simulink library "ComponentsLib"  (R2022b)
settings: Solver=VariableStepAuto  StartTime=0.0  StopTime=10.0  RelTol=1e-3
undefined symbols (not defined in the file or in its folder): SimIn, SimPar
libraries: simulink_extras x23, libAxisTransformations x2
settings Model: Creator=tbritton  LastModifiedBy=macheson
settings SolverCC: AlgebraicLoopSolver=TrustRegion
settings DebuggingCC: UnconnectedInputMsg=warning  UnconnectedOutputMsg=warning  UnconnectedLineMsg=warning  SFMachineParentedDataDiag=warning
settings ModelReferenceCC: EnableRefExpFcnMdlSchedulingChecks=on
settings RTWCC: DLArmComputeVersion=19.05

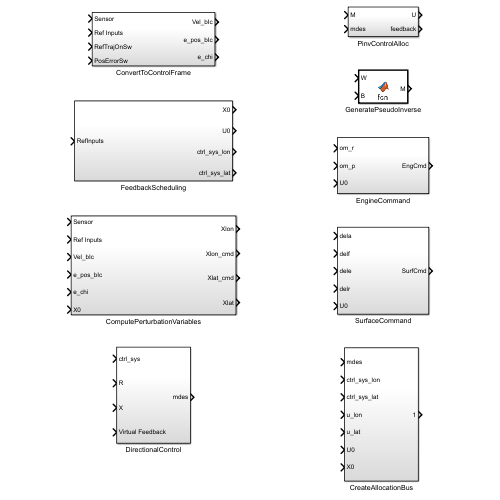
[thumbnail: Simulink's stored preview of the top-level diagram]
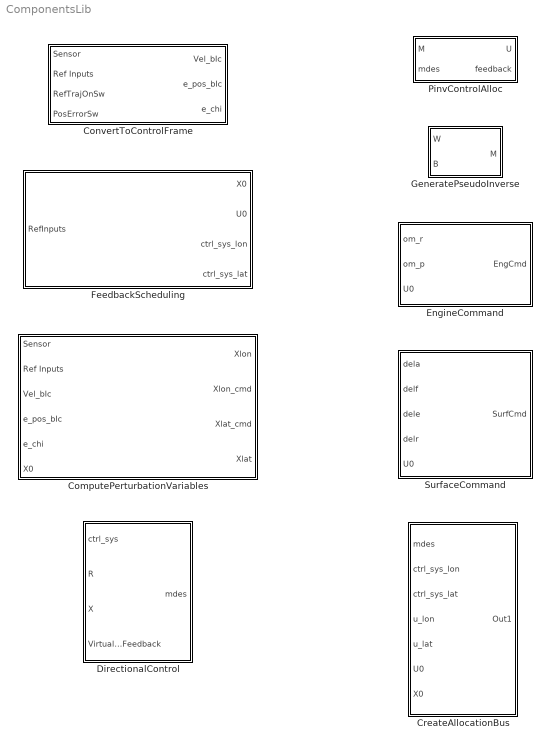
== system ComponentsLib ==
  ComputePerturbationVariables : Subsystem
  ConvertToControlFrame : Subsystem
  CreateAllocationBus : Subsystem
  DirectionalControl : Subsystem
  EngineCommand : Subsystem
  FeedbackScheduling : Subsystem
  GeneratePseudoInverse : MATLAB Function  TreatAsAtomicUnit=on
  PinvControlAlloc : Subsystem
  SurfaceCommand : Subsystem

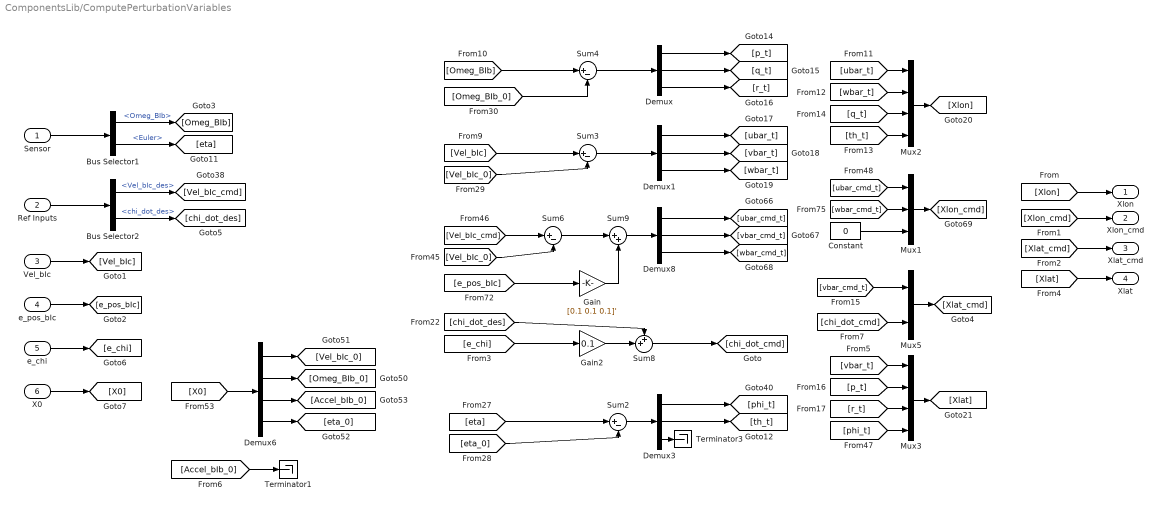
== system ComponentsLib/ComputePerturbationVariables ==
  Sensor : Inport  OutDataTypeStr=Bus: SensorBus
  Ref Inputs : Inport  Port=2  OutDataTypeStr=Bus: BUS_REF_INPUT
  Vel_bIc : Inport  Port=3
  e_pos_bIc : Inport  Port=4
  e_chi : Inport  Port=5
  X0 : Inport  Port=6
  Bus Selector1 : BusSelector  OutputSignals=Omeg_BIb,Euler
  Bus Selector2 : BusSelector  OutputSignals=Vel_bIc_des,chi_dot_des
  Constant : Constant  Value=0
  Demux{,1,3,8} (4 alike) : Demux  Outputs=3
  Demux6 : Demux  Outputs=[3 3 3 3]
  Gain : Gain  Gain=[0.1 0.1 0.1]'
  Gain2 : Gain  Gain=0.1
  Mux1 : Mux  Inputs=3
  Mux2 : Mux
  Mux3 : Mux
  Mux5 : Mux  Inputs=2
  Sum{2..4,6} (4 alike) : Sum  Inputs=|+-
  Sum8 : Sum  Inputs=++|
  Sum9 : Sum  Inputs=|++
  Terminator1 : Terminator
  Terminator3 : Terminator
  Xlon : Outport
  Xlon_cmd : Outport  Port=2
  Xlat_cmd : Outport  Port=3
  Xlat : Outport  Port=4
  wires:
  [Omeg_BIb_0] -> Sum4/2
  Sum9/1 -> Demux8/1
  [Vel_bIc] -> Sum3/1
  [Vel_bIc_0] -> Sum3/2
  [chi_dot_cmd] -> Mux5/2
  Demux1/1 -> [ubar_t]
  [eta] -> Sum2/1
  Demux3/2 -> [th_t]
  Demux3/3 -> Terminator3/1
  Demux3/1 -> [phi_t]
  Demux1/3 -> [wbar_t]
  Demux/1 -> [p_t]
  Gain2/1 -> Sum8/2
  Mux2/1 -> [Xlon]
  Sum8/1 -> [chi_dot_cmd]
  [e_chi] -> Gain2/1
  [Vel_bIc_0] -> Sum6/2
  [r_t] -> Mux3/3
  [vbar_cmd_t] -> Mux5/1
  Gain/1 -> Sum9/2
  [ubar_t] -> Mux2/1
  Mux5/1 -> [Xlat_cmd]
  [q_t] -> Mux2/3
  Demux1/2 -> [vbar_t]
  [chi_dot_des] -> Sum8/1
  Mux1/1 -> [Xlon_cmd]
  [vbar_t] -> Mux3/1
  [wbar_cmd_t] -> Mux1/2
  [e_pos_bIc] -> Gain/1
  Demux8/3 -> [wbar_cmd_t]
  Constant/1 -> Mux1/3
  [phi_t] -> Mux3/4
  Demux8/1 -> [ubar_cmd_t]
  Sum6/1 -> Sum9/1
  [Vel_bIc_cmd] -> Sum6/1
  Demux8/2 -> [vbar_cmd_t]
  Sum2/1 -> Demux3/1
  Demux/3 -> [r_t]
  Sum3/1 -> Demux1/1
  Sum4/1 -> Demux/1
  Mux3/1 -> [Xlat]
  [p_t] -> Mux3/2
  [th_t] -> Mux2/4
  Demux/2 -> [q_t]
  [ubar_cmd_t] -> Mux1/1
  [wbar_t] -> Mux2/2
  [eta_0] -> Sum2/2
  [Omeg_BIb] -> Sum4/1
  [Xlon] -> Xlon/1
  [Xlon_cmd] -> Xlon_cmd/1
  [Xlat_cmd] -> Xlat_cmd/1
  [Xlat] -> Xlat/1
  Bus Selector1/2 -> [eta]  "<Euler>"
  Sensor/1 -> Bus Selector1/1
  Bus Selector1/1 -> [Omeg_BIb]  "<Omeg_BIb>"
  Vel_bIc/1 -> [Vel_bIc]
  Ref Inputs/1 -> Bus Selector2/1
  Bus Selector2/1 -> [Vel_bIc_cmd]  "<Vel_bIc_des>"
  Bus Selector2/2 -> [chi_dot_des]  "<chi_dot_des>"
  e_pos_bIc/1 -> [e_pos_bIc]
  e_chi/1 -> [e_chi]
  Demux6/1 -> [Vel_bIc_0]
  Demux6/3 -> [Accel_bIb_0]
  [X0] -> Demux6/1
  Demux6/4 -> [eta_0]
  Demux6/2 -> [Omeg_BIb_0]
  X0/1 -> [X0]
  [Accel_bIb_0] -> Terminator1/1

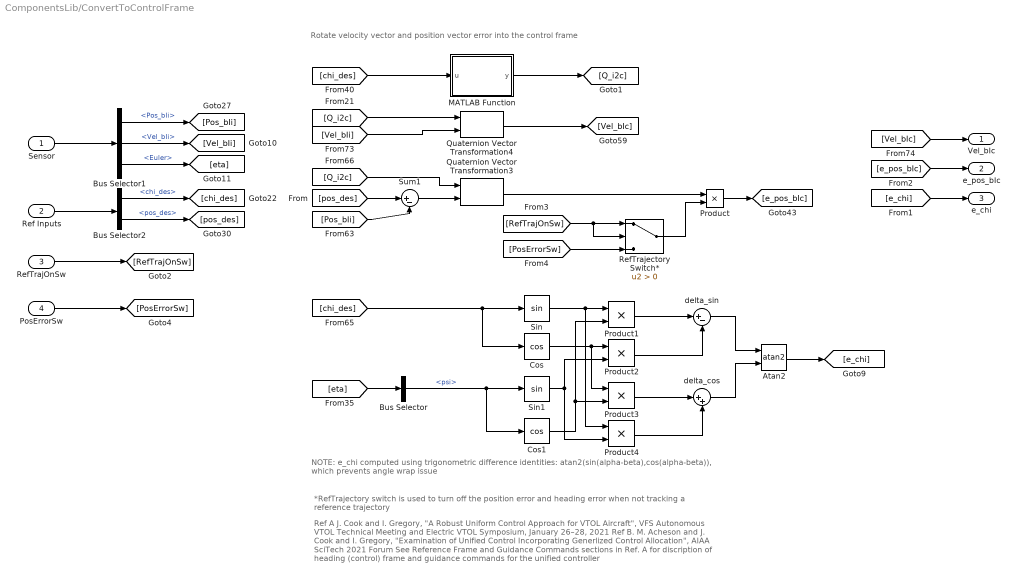
== system ComponentsLib/ConvertToControlFrame ==
  note: NOTE: e_chi computed using trigonometric difference identities: atan2(sin(alpha-beta),cos(alpha-beta)), which prevents angle wrap issue
  note: *RefTrajectory switch is used to turn off the position error and heading error when not tracking a reference trajectory
  note: Ref A
      | J. Cook and I. Gregory, "A Robust Uniform Control Approach for VTOL Aircraft", VFS Autonomous VTOL Technical Meeting and Electric VTOL Symposium, January 26–28, 2021
      |
      | Ref B.
      | M. Acheson and J. Cook and I. Gregory, "Examination of Unified Control Incorporating Generlized Control Allocation", AIAA SciTech 2021 Forum
      |
      | See Reference Frame and Guidance Commands sections in Ref. A for discription of heading (control) frame and guidance commands for the unified controller
  note: Rotate velocity vector and position vector error into the control frame
  Sensor : Inport  OutDataTypeStr=Bus: SensorBus
  Ref Inputs : Inport  Port=2  OutDataTypeStr=Bus: BUS_REF_INPUT
  RefTrajOnSw : Inport  Port=3
  PosErrorSw : Inport  Port=4
  Atan2 : Trigonometry  Operator=atan2
  Bus Selector : BusSelector  OutputSignals=psi
  Bus Selector1 : BusSelector  OutputSignals=Pos_bIi,Vel_bIi,Euler
  Bus Selector2 : BusSelector  OutputSignals=chi_des,pos_des
  Cos : Trigonometry  Operator=cos
  Cos1 : Trigonometry  Operator=cos
  MATLAB Function : MATLAB Function  TreatAsAtomicUnit=on
  Product{,1..4} (5 alike) : Product
  Quaternion Vector Transformation3 : libAxisTransformations/Quaternion Vector Transformation  n=0
  Quaternion Vector Transformation4 : libAxisTransformations/Quaternion Vector Transformation  n=0
  RefTrajectory Switch* : Switch  Criteria=u2 > Threshold  SaturateOnIntegerOverflow=off  InputSameDT=off
  Sin : Trigonometry
  Sin1 : Trigonometry
  Sum1 : Sum  Inputs=|+-
  delta_cos : Sum  Inputs=|++
  delta_sin : Sum  Inputs=|+-
  Vel_bIc : Outport
  e_pos_bIc : Outport  Port=2
  e_chi : Outport  Port=3
  wires:
  Sensor/1 -> Bus Selector1/1
  Quaternion Vector Transformation4/1 -> [Vel_bIc]
  [chi_des] -> Cos/1, Sin/1
  Sum1/1 -> Quaternion Vector Transformation3/2
  [e_pos_bIc] -> e_pos_bIc/1
  RefTrajOnSw/1 -> [RefTrajOnSw]
  Bus Selector2/1 -> [chi_des]  "<chi_des>"
  Bus Selector1/2 -> [Vel_bIi]  "<Vel_bIi>"
  PosErrorSw/1 -> [PosErrorSw]
  [Vel_bIi] -> Quaternion Vector Transformation4/2
  Atan2/1 -> [e_chi]
  Bus Selector1/1 -> [Pos_bIi]  "<Pos_bIi>"
  Bus Selector2/2 -> [pos_des]  "<pos_des>"
  [RefTrajOnSw] -> RefTrajectory Switch*/1, RefTrajectory Switch*/2
  [Vel_bIc] -> Vel_bIc/1
  [Pos_bIi] -> Sum1/2
  RefTrajectory Switch*/1 -> Product/2
  [chi_des] -> MATLAB Function/1(u)
  [e_chi] -> e_chi/1
  [pos_des] -> Sum1/1
  Quaternion Vector Transformation3/1 -> Product/1
  [Q_i2c] -> Quaternion Vector Transformation3/1
  Product/1 -> [e_pos_bIc]
  Ref Inputs/1 -> Bus Selector2/1
  MATLAB Function/1(y) -> [Q_i2c]
  Bus Selector1/3 -> [eta]  "<Euler>"
  [PosErrorSw] -> RefTrajectory Switch*/3
  [eta] -> Bus Selector/1
  [Q_i2c] -> Quaternion Vector Transformation4/1
  Bus Selector/1 -> Cos1/1, Sin1/1  "<psi>"
  Sin/1 -> Product1/1, Product4/1
  Cos/1 -> Product3/1, Product2/1
  Sin1/1 -> Product4/2, Product2/2
  Cos1/1 -> Product3/2, Product1/2
  Product1/1 -> delta_sin/1
  Product2/1 -> delta_sin/2
  Product3/1 -> delta_cos/1
  Product4/1 -> delta_cos/2
  delta_sin/1 -> Atan2/1
  delta_cos/1 -> Atan2/2

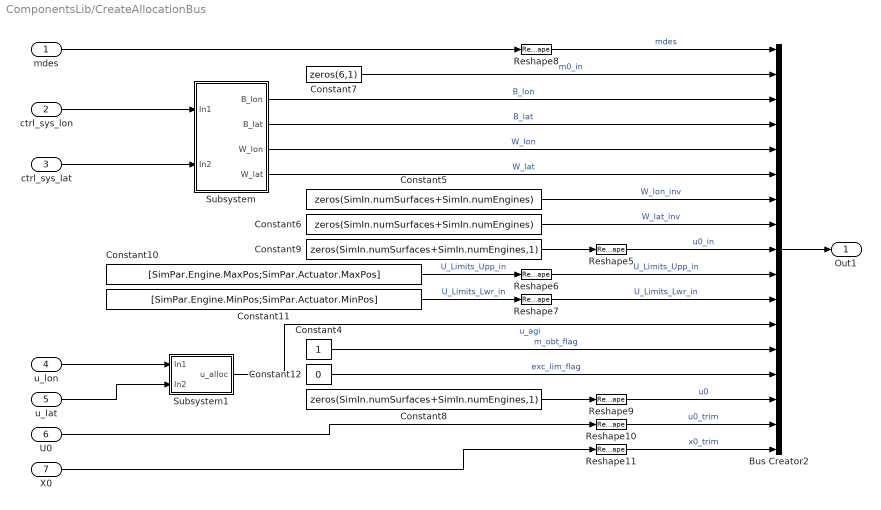
== system ComponentsLib/CreateAllocationBus ==
  mdes : Inport
  ctrl_sys_lon : Inport  Port=2
  ctrl_sys_lat : Inport  Port=3
  u_lon : Inport  Port=4
  u_lat : Inport  Port=5
  U0 : Inport  Port=6
  X0 : Inport  Port=7
  Bus Creator2 : BusCreator  Inputs=17  OutDataTypeStr=Bus: BUS_ALLOC
  Constant10 : Constant  Value=[SimPar.Engine.MaxPos;SimPar.Actuator.MaxPos]
  Constant11 : Constant  Value=[SimPar.Engine.MinPos;SimPar.Actuator.MinPos]
  Constant12 : Constant  Value=0
  Constant4 : Constant
  Constant5 : Constant  Value=zeros(SimIn.numSurfaces+SimIn.numEngines)
  Constant6 : Constant  Value=zeros(SimIn.numSurfaces+SimIn.numEngines)
  Constant7 : Constant  Value=zeros(6,1)
  Constant8 : Constant  Value=zeros(SimIn.numSurfaces+SimIn.numEngines,1)
  Constant9 : Constant  Value=zeros(SimIn.numSurfaces+SimIn.numEngines,1)
  Reshape{5..11} (7 alike) : Reshape
  Subsystem : Subsystem
  Subsystem1 : Subsystem
  Out1 : Outport
  wires:
  Constant6/1 -> Bus Creator2/8  "W_lat_inv"
  Constant7/1 -> Bus Creator2/2  "m0_in"
  Constant5/1 -> Bus Creator2/7  "W_lon_inv"
  Subsystem/2(B_lat) -> Bus Creator2/4  "B_lat"
  Subsystem/4(W_lat) -> Bus Creator2/6  "W_lat"
  Constant10/1 -> Reshape6/1  "U_Limits_Upp_in"
  Reshape8/1 -> Bus Creator2/1  "mdes"
  u_lat/1 -> Subsystem1/2(In2)
  Constant12/1 -> Bus Creator2/14  "exc_lim_flag"
  Constant9/1 -> Reshape5/1
  Subsystem/1(B_lon) -> Bus Creator2/3  "B_lon"
  Subsystem/3(W_lon) -> Bus Creator2/5  "W_lon"
  Constant11/1 -> Reshape7/1  "U_Limits_Lwr_in"
  Reshape10/1 -> Bus Creator2/16  "u0_trim"
  Constant8/1 -> Reshape9/1
  Reshape7/1 -> Bus Creator2/11  "U_Limits_Lwr_in"
  U0/1 -> Reshape10/1
  Constant4/1 -> Bus Creator2/13  "m_obt_flag"
  Subsystem1/1(u_alloc) -> Bus Creator2/12  "u_agi"
  Reshape9/1 -> Bus Creator2/15  "u0"
  Reshape11/1 -> Bus Creator2/17  "x0_trim"
  Reshape6/1 -> Bus Creator2/10  "U_Limits_Upp_in"
  Reshape5/1 -> Bus Creator2/9  "u0_in"
  ctrl_sys_lon/1 -> Subsystem/1(In1)
  u_lon/1 -> Subsystem1/1(In1)
  X0/1 -> Reshape11/1
  Bus Creator2/1 -> Out1/1
  ctrl_sys_lat/1 -> Subsystem/2(In2)
  mdes/1 -> Reshape8/1

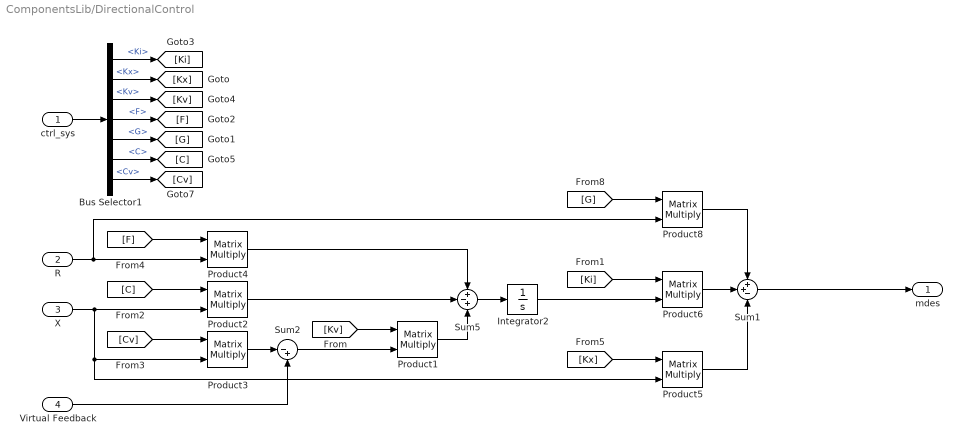
== system ComponentsLib/DirectionalControl ==
  ctrl_sys : Inport
  R : Inport  Port=2
  X : Inport  Port=3
  Virtual Feedback : Inport  Port=4
  Bus Selector1 : BusSelector  OutputSignals=Ki,Kx,Kv,F,G,C,Cv
  Integrator2 : Integrator  UpperSaturationLimit=[10 10 1]  LowerSaturationLimit=[-10 -10 -1]
  Product{1..6,8} (7 alike) : Product  Multiplication=Matrix(*)
  Sum1 : Sum  Inputs=++-
  Sum2 : Sum  Inputs=|-+
  Sum5 : Sum  Inputs=+-+
  mdes : Outport
  wires:
  Sum1/1 -> mdes/1
  X/1 -> Product2/2, Product3/2, Product5/2
  [C] -> Product2/1
  Product2/1 -> Sum5/2
  R/1 -> Product8/2, Product4/2
  Sum5/1 -> Integrator2/1
  ctrl_sys/1 -> Bus Selector1/1
  [Cv] -> Product3/1
  Product3/1 -> Sum2/1
  Integrator2/1 -> Product6/2
  Sum2/1 -> Product1/2
  [Kv] -> Product1/1
  Product1/1 -> Sum5/3
  [Ki] -> Product6/1
  Product6/1 -> Sum1/2
  [Kx] -> Product5/1
  Product5/1 -> Sum1/3
  [F] -> Product4/1
  Product4/1 -> Sum5/1
  Product8/1 -> Sum1/1
  [G] -> Product8/1
  Virtual Feedback/1 -> Sum2/2
  Bus Selector1/7 -> [Cv]  "<Cv>"
  Bus Selector1/6 -> [C]  "<C>"
  Bus Selector1/5 -> [G]  "<G>"
  Bus Selector1/4 -> [F]  "<F>"
  Bus Selector1/3 -> [Kv]  "<Kv>"
  Bus Selector1/2 -> [Kx]  "<Kx>"
  Bus Selector1/1 -> [Ki]  "<Ki>"

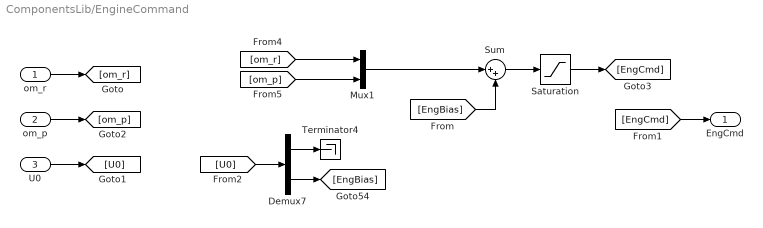
== system ComponentsLib/EngineCommand ==
  om_r : Inport
  om_p : Inport  Port=2
  U0 : Inport  Port=3
  Demux7 : Demux  Outputs=[-1 9]
  Mux1 : Mux  Inputs=2
  Saturation : Saturate  UpperLimit=SimPar.Engine.MaxPos  LowerLimit=SimPar.Engine.MinPos
  Sum : Sum  Inputs=|++
  Terminator4 : Terminator
  EngCmd : Outport
  wires:
  Mux1/1 -> Sum/1
  Sum/1 -> Saturation/1
  [EngBias] -> Sum/2
  U0/1 -> [U0]
  om_r/1 -> [om_r]
  om_p/1 -> [om_p]
  [om_r] -> Mux1/1
  [om_p] -> Mux1/2
  Demux7/2 -> [EngBias]
  [U0] -> Demux7/1
  Demux7/1 -> Terminator4/1
  Saturation/1 -> [EngCmd]
  [EngCmd] -> EngCmd/1

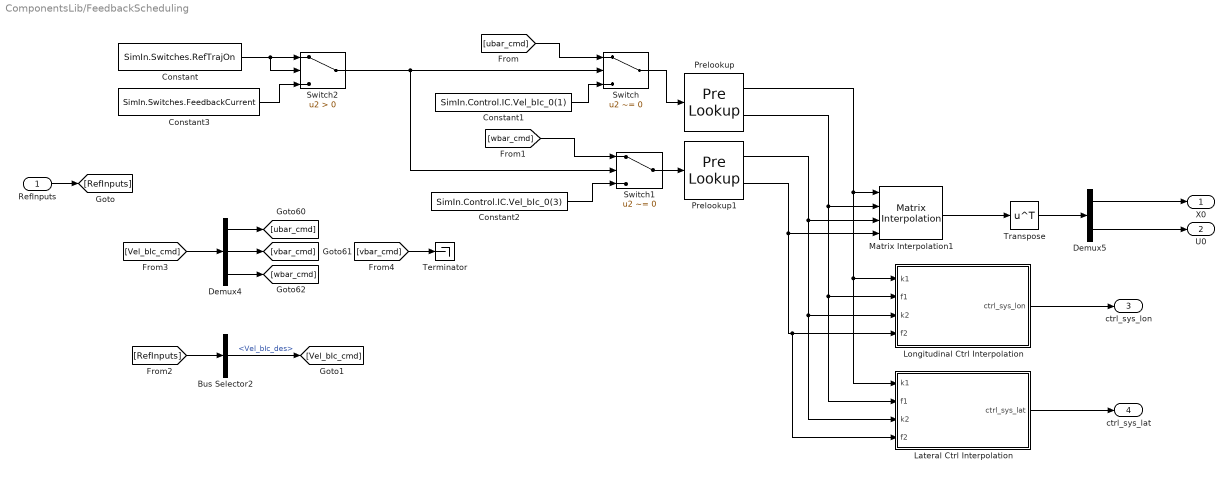
== system ComponentsLib/FeedbackScheduling ==
  RefInputs : Inport  OutDataTypeStr=Bus: BUS_REF_INPUT
  Bus Selector2 : BusSelector  OutputSignals=Vel_bIc_des
  Constant : Constant  Value=SimIn.Switches.RefTrajOn
  Constant1 : Constant  Value=SimIn.Control.IC.Vel_bIc_0(1)
  Constant2 : Constant  Value=SimIn.Control.IC.Vel_bIc_0(3)
  Constant3 : Constant  Value=SimIn.Switches.FeedbackCurrent
  Demux4 : Demux  Outputs=3
  Demux5 : Demux  Outputs=[12 13]
  Lateral Ctrl Interpolation : Subsystem
  Longitudinal Ctrl Interpolation : Subsystem
  Matrix Interpolation1 : simulink_extras/Additional Lookup Tables/Matrix Interpolation  InterpMethod=Linear  ExtrapMethod=Clip  InterpolateDimension=2  TableData=SimIn.Control.trim.XU0_interp  SimulateUsing=Code generation
  Prelookup : PreLookup  BreakpointsData=SimIn.Control.trim.UH
  Prelookup1 : PreLookup  BreakpointsData=SimIn.Control.trim.WH
  Switch : Switch  Criteria=u2 ~= 0  SaturateOnIntegerOverflow=off  InputSameDT=off
  Switch1 : Switch  Criteria=u2 ~= 0  SaturateOnIntegerOverflow=off  InputSameDT=off
  Switch2 : Switch  Criteria=u2 > Threshold  SaturateOnIntegerOverflow=off  InputSameDT=off
  Terminator : Terminator
  Transpose : Math  Operator=transpose
  X0 : Outport
  U0 : Outport  Port=2
  ctrl_sys_lon : Outport  Port=3
  ctrl_sys_lat : Outport  Port=4
  wires:
  Constant3/1 -> Switch2/3
  Constant/1 -> Switch2/2, Switch2/1
  Switch2/1 -> Switch/2, Switch1/2
  Constant2/1 -> Switch1/3
  Switch1/1 -> Prelookup1/1
  Switch/1 -> Prelookup/1
  Constant1/1 -> Switch/3
  Longitudinal Ctrl Interpolation/1(ctrl_sys_lon) -> ctrl_sys_lon/1
  Lateral Ctrl Interpolation/1(ctrl_sys_lat) -> ctrl_sys_lat/1
  Prelookup1/2 -> Matrix Interpolation1/4, Lateral Ctrl Interpolation/4(f2), Longitudinal Ctrl Interpolation/4(f2)
  Prelookup1/1 -> Matrix Interpolation1/3, Lateral Ctrl Interpolation/3(k2), Longitudinal Ctrl Interpolation/3(k2)
  [wbar_cmd] -> Switch1/1
  Demux5/2 -> U0/1
  Demux5/1 -> X0/1
  Transpose/1 -> Demux5/1
  Matrix Interpolation1/1 -> Transpose/1
  Prelookup/1 -> Lateral Ctrl Interpolation/1(k1), Longitudinal Ctrl Interpolation/1(k1), Matrix Interpolation1/1
  Prelookup/2 -> Matrix Interpolation1/2, Lateral Ctrl Interpolation/2(f1), Longitudinal Ctrl Interpolation/2(f1)
  Demux4/1 -> [ubar_cmd]
  Demux4/3 -> [wbar_cmd]
  Demux4/2 -> [vbar_cmd]
  [Vel_bIc_cmd] -> Demux4/1
  RefInputs/1 -> [RefInputs]
  [ubar_cmd] -> Switch/1
  [RefInputs] -> Bus Selector2/1
  Bus Selector2/1 -> [Vel_bIc_cmd]  "<Vel_bIc_des>"
  [vbar_cmd] -> Terminator/1

== system ComponentsLib/PinvControlAlloc ==
  M : Inport
  mdes : Inport  Port=2
  Demux : Demux  Outputs=[-1 1]
  Product7 : Product  Multiplication=Matrix(*)
  U : Outport
  feedback : Outport  Port=2
  wires:
  Product7/1 -> Demux/1
  M/1 -> Product7/1
  Demux/2 -> feedback/1
  mdes/1 -> Product7/2
  Demux/1 -> U/1

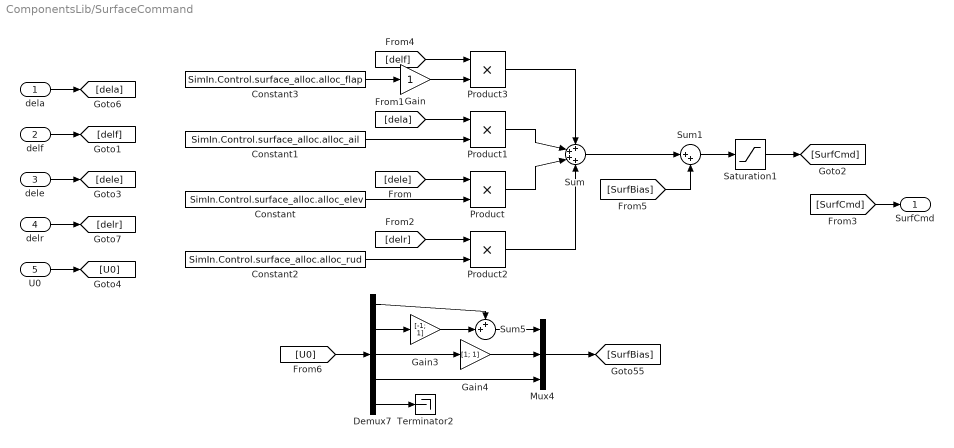
== system ComponentsLib/SurfaceCommand ==
  dela : Inport
  delf : Inport  Port=2
  dele : Inport  Port=3
  delr : Inport  Port=4
  U0 : Inport  Port=5
  Constant : Constant  Value=SimIn.Control.surface_alloc.alloc_elev
  Constant1 : Constant  Value=SimIn.Control.surface_alloc.alloc_ail
  Constant2 : Constant  Value=SimIn.Control.surface_alloc.alloc_rud
  Constant3 : Constant  Value=SimIn.Control.surface_alloc.alloc_flap
  Demux7 : Demux  Outputs=[1 1 1 1 -1]
  Gain : Gain
  Gain3 : Gain  Gain=[-1; 1]
  Gain4 : Gain  Gain=[1; 1]
  Mux4 : Mux  Inputs=3
  Product{,1..3} (4 alike) : Product
  Saturation1 : Saturate  UpperLimit=SimPar.Actuator.MaxPos  LowerLimit=SimPar.Actuator.MinPos
  Sum : Sum  Inputs=++++
  Sum1 : Sum  Inputs=|++
  Sum5 : Sum  Inputs=++|
  Terminator2 : Terminator
  SurfCmd : Outport
  wires:
  Gain/1 -> Product3/2
  [delf] -> Product3/1
  Constant3/1 -> Gain/1
  Product3/1 -> Sum/1
  [SurfBias] -> Sum1/2
  Sum/1 -> Sum1/1
  Sum1/1 -> Saturation1/1
  Product2/1 -> Sum/4
  Product1/1 -> Sum/2
  Product/1 -> Sum/3
  Constant2/1 -> Product2/2
  [delr] -> Product2/1
  Constant1/1 -> Product1/2
  [dela] -> Product1/1
  Constant/1 -> Product/2
  [dele] -> Product/1
  U0/1 -> [U0]
  Gain4/1 -> Mux4/2
  Demux7/1 -> Sum5/1
  Demux7/5 -> Terminator2/1
  Gain3/1 -> Sum5/2
  Demux7/3 -> Gain4/1
  Demux7/4 -> Mux4/3
  [U0] -> Demux7/1
  Mux4/1 -> [SurfBias]
  Demux7/2 -> Gain3/1
  Sum5/1 -> Mux4/1
  Saturation1/1 -> [SurfCmd]
  [SurfCmd] -> SurfCmd/1
  delf/1 -> [delf]
  delr/1 -> [delr]
  dela/1 -> [dela]
  dele/1 -> [dele]

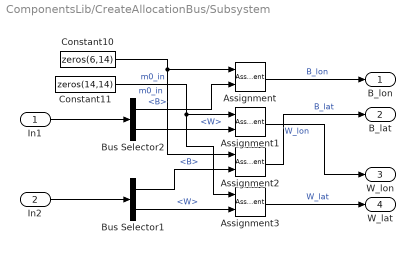
== system ComponentsLib/CreateAllocationBus/Subsystem ==
  In1 : Inport
  In2 : Inport  Port=2
  Assignment : Assignment  NumberOfDimensions=2  DiagnosticForDimensions=Warning  IndexOptions=Index vector (dialog),Index vector (dialog)  Indices=1:3,1:12  OutputSizes=1,1
  Assignment1 : Assignment  NumberOfDimensions=2  DiagnosticForDimensions=Warning  IndexOptions=Index vector (dialog),Index vector (dialog)  Indices=1:12,1:12  OutputSizes=1,1
  Assignment2 : Assignment  NumberOfDimensions=2  DiagnosticForDimensions=Warning  IndexOptions=Index vector (dialog),Index vector (dialog)  Indices=1:3,1:11  OutputSizes=1,1
  Assignment3 : Assignment  NumberOfDimensions=2  DiagnosticForDimensions=Warning  IndexOptions=Index vector (dialog),Index vector (dialog)  Indices=1:11,1:11  OutputSizes=1,1
  Bus Selector1 : BusSelector  OutputSignals=B,W
  Bus Selector2 : BusSelector  OutputSignals=B,W
  Constant10 : Constant  Value=zeros(6,14)
  Constant11 : Constant  Value=zeros(14,14)
  B_lon : Outport
  B_lat : Outport  Port=2
  W_lon : Outport  Port=3
  W_lat : Outport  Port=4
  wires:
  In2/1 -> Bus Selector1/1
  Assignment/1 -> B_lon/1  "B_lon"
  Assignment3/1 -> W_lat/1  "W_lat"
  Assignment2/1 -> B_lat/1  "B_lat"
  In1/1 -> Bus Selector2/1
  Constant11/1 -> Assignment1/1, Assignment3/1  "m0_in"
  Constant10/1 -> Assignment/1, Assignment2/1  "m0_in"
  Assignment1/1 -> W_lon/1  "W_lon"
  Bus Selector1/2 -> Assignment3/2  "<W>"
  Bus Selector1/1 -> Assignment2/2  "<B>"
  Bus Selector2/2 -> Assignment1/2  "<W>"
  Bus Selector2/1 -> Assignment/2  "<B>"

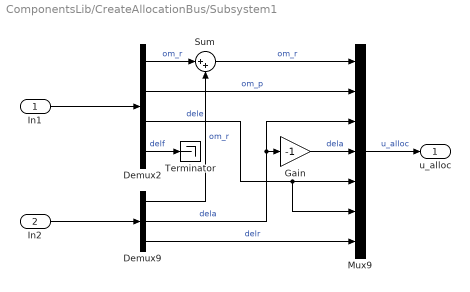
== system ComponentsLib/CreateAllocationBus/Subsystem1 ==
  In1 : Inport
  In2 : Inport  Port=2
  Demux2 : Demux  Outputs=[8 1 1 1]
  Demux9 : Demux  Outputs=[8 1 1]
  Gain : Gain  Gain=-1
  Mux9 : Mux  Inputs=7
  Sum : Sum  Inputs=|++
  Terminator : Terminator
  u_alloc : Outport
  wires:
  Gain/1 -> Mux9/4  "dela"
  In1/1 -> Demux2/1
  Mux9/1 -> u_alloc/1  "u_alloc"
  Demux9/2 -> Mux9/3, Gain/1  "dela"
  Demux2/1 -> Sum/1  "om_r"
  Sum/1 -> Mux9/1  "om_r"
  Demux2/2 -> Mux9/2  "om_p"
  Demux2/3 -> Mux9/6, Mux9/5  "dele"
  Demux2/4 -> Terminator/1  "delf"
  In2/1 -> Demux9/1
  Demux9/3 -> Mux9/7  "delr"
  Demux9/1 -> Sum/2  "om_r"

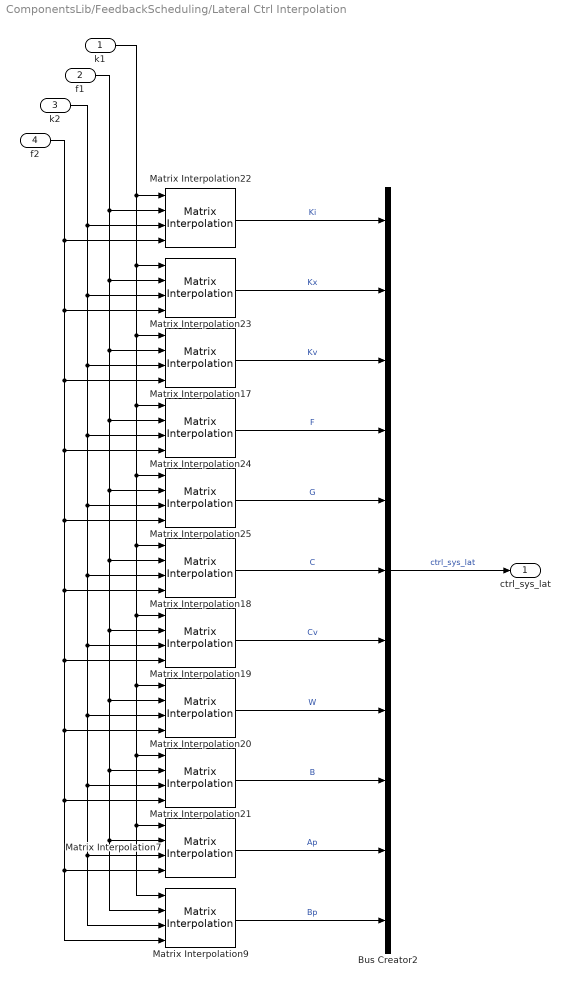
== system ComponentsLib/FeedbackScheduling/Lateral Ctrl Interpolation ==
  k1 : Inport
  f1 : Inport  Port=2
  k2 : Inport  Port=3
  f2 : Inport  Port=4
  Bus Creator2 : BusCreator  Inputs=11
  Matrix Interpolation17 : simulink_extras/Additional Lookup Tables/Matrix Interpolation  InterpMethod=Linear  ExtrapMethod=Clip  InterpolateDimension=2  TableData=SimIn.Control.trim.Kv_lat_interp  SimulateUsing=Code generation
  Matrix Interpolation18 : simulink_extras/Additional Lookup Tables/Matrix Interpolation  InterpMethod=Linear  ExtrapMethod=Clip  InterpolateDimension=2  TableData=SimIn.Control.trim.C_lat_interp  SimulateUsing=Code generation
  Matrix Interpolation19 : simulink_extras/Additional Lookup Tables/Matrix Interpolation  InterpMethod=Linear  ExtrapMethod=Clip  InterpolateDimension=2  TableData=SimIn.Control.trim.Cv_lat_interp  SimulateUsing=Code generation
  Matrix Interpolation20 : simulink_extras/Additional Lookup Tables/Matrix Interpolation  InterpMethod=Linear  ExtrapMethod=Clip  InterpolateDimension=2  TableData=SimIn.Control.trim.W_lat_interp  SimulateUsing=Code generation
  Matrix Interpolation21 : simulink_extras/Additional Lookup Tables/Matrix Interpolation  InterpMethod=Linear  ExtrapMethod=Clip  InterpolateDimension=2  TableData=SimIn.Control.trim.B_lat_interp  SimulateUsing=Code generation
  Matrix Interpolation22 : simulink_extras/Additional Lookup Tables/Matrix Interpolation  InterpMethod=Linear  ExtrapMethod=Clip  InterpolateDimension=2  TableData=SimIn.Control.trim.Ki_lat_interp  SimulateUsing=Code generation
  Matrix Interpolation23 : simulink_extras/Additional Lookup Tables/Matrix Interpolation  InterpMethod=Linear  ExtrapMethod=Clip  InterpolateDimension=2  TableData=SimIn.Control.trim.Kx_lat_interp  SimulateUsing=Code generation
  Matrix Interpolation24 : simulink_extras/Additional Lookup Tables/Matrix Interpolation  InterpMethod=Linear  ExtrapMethod=Clip  InterpolateDimension=2  TableData=SimIn.Control.trim.F_lat_interp  SimulateUsing=Code generation
  Matrix Interpolation25 : simulink_extras/Additional Lookup Tables/Matrix Interpolation  InterpMethod=Linear  ExtrapMethod=Clip  InterpolateDimension=2  TableData=SimIn.Control.trim.G_lat_interp  SimulateUsing=Code generation
  Matrix Interpolation7 : simulink_extras/Additional Lookup Tables/Matrix Interpolation  InterpMethod=Linear  ExtrapMethod=Clip  InterpolateDimension=2  TableData=SimIn.Control.trim.Ap_lat_interp  SimulateUsing=Code generation
  Matrix Interpolation9 : simulink_extras/Additional Lookup Tables/Matrix Interpolation  InterpMethod=Linear  ExtrapMethod=Clip  InterpolateDimension=2  TableData=SimIn.Control.trim.Bp_lat_interp  SimulateUsing=Code generation
  ctrl_sys_lat : Outport
  wires:
  Bus Creator2/1 -> ctrl_sys_lat/1  "ctrl_sys_lat"
  Matrix Interpolation7/1 -> Bus Creator2/10  "Ap"
  Matrix Interpolation21/1 -> Bus Creator2/9  "B"
  Matrix Interpolation24/1 -> Bus Creator2/4  "F"
  Matrix Interpolation25/1 -> Bus Creator2/5  "G"
  Matrix Interpolation9/1 -> Bus Creator2/11  "Bp"
  Matrix Interpolation23/1 -> Bus Creator2/2  "Kx"
  Matrix Interpolation19/1 -> Bus Creator2/7  "Cv"
  Matrix Interpolation18/1 -> Bus Creator2/6  "C"
  Matrix Interpolation17/1 -> Bus Creator2/3  "Kv"
  Matrix Interpolation22/1 -> Bus Creator2/1  "Ki"
  f1/1 -> Matrix Interpolation9/2, Matrix Interpolation7/2, Matrix Interpolation21/2, Matrix Interpolation20/2, Matrix Interpolation19/2, Matrix Interpolation18/2, Matrix Interpolation25/2, Matrix Interpolation24/2, Matrix Interpolation17/2, Matrix Interpolation23/2, Matrix Interpolation22/2
  f2/1 -> Matrix Interpolation9/4, Matrix Interpolation7/4, Matrix Interpolation21/4, Matrix Interpolation20/4, Matrix Interpolation19/4, Matrix Interpolation18/4, Matrix Interpolation25/4, Matrix Interpolation24/4, Matrix Interpolation17/4, Matrix Interpolation23/4, Matrix Interpolation22/4
  Matrix Interpolation20/1 -> Bus Creator2/8  "W"
  k2/1 -> Matrix Interpolation9/3, Matrix Interpolation7/3, Matrix Interpolation21/3, Matrix Interpolation20/3, Matrix Interpolation19/3, Matrix Interpolation18/3, Matrix Interpolation25/3, Matrix Interpolation24/3, Matrix Interpolation17/3, Matrix Interpolation23/3, Matrix Interpolation22/3
  k1/1 -> Matrix Interpolation24/1, Matrix Interpolation20/1, Matrix Interpolation7/1, Matrix Interpolation9/1, Matrix Interpolation21/1, Matrix Interpolation19/1, Matrix Interpolation18/1, Matrix Interpolation25/1, Matrix Interpolation17/1, Matrix Interpolation23/1, Matrix Interpolation22/1

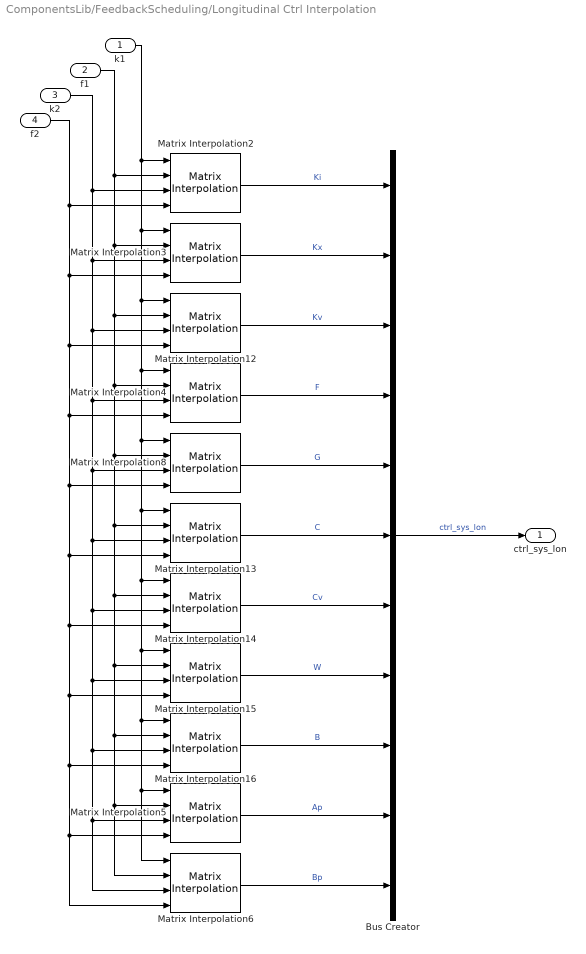
== system ComponentsLib/FeedbackScheduling/Longitudinal Ctrl Interpolation ==
  k1 : Inport
  f1 : Inport  Port=2
  k2 : Inport  Port=3
  f2 : Inport  Port=4
  Bus Creator : BusCreator  Inputs=11
  Matrix Interpolation12 : simulink_extras/Additional Lookup Tables/Matrix Interpolation  InterpMethod=Linear  ExtrapMethod=Clip  InterpolateDimension=2  TableData=SimIn.Control.trim.Kv_lon_interp  SimulateUsing=Code generation
  Matrix Interpolation13 : simulink_extras/Additional Lookup Tables/Matrix Interpolation  InterpMethod=Linear  ExtrapMethod=Clip  InterpolateDimension=2  TableData=SimIn.Control.trim.C_lon_interp  SimulateUsing=Code generation
  Matrix Interpolation14 : simulink_extras/Additional Lookup Tables/Matrix Interpolation  InterpMethod=Linear  ExtrapMethod=Clip  InterpolateDimension=2  TableData=SimIn.Control.trim.Cv_lon_interp  SimulateUsing=Code generation
  Matrix Interpolation15 : simulink_extras/Additional Lookup Tables/Matrix Interpolation  InterpMethod=Linear  ExtrapMethod=Clip  InterpolateDimension=2  TableData=SimIn.Control.trim.W_lon_interp  SimulateUsing=Code generation
  Matrix Interpolation16 : simulink_extras/Additional Lookup Tables/Matrix Interpolation  InterpMethod=Linear  ExtrapMethod=Clip  InterpolateDimension=2  TableData=SimIn.Control.trim.B_lon_interp  SimulateUsing=Code generation
  Matrix Interpolation2 : simulink_extras/Additional Lookup Tables/Matrix Interpolation  InterpMethod=Linear  ExtrapMethod=Clip  InterpolateDimension=2  TableData=SimIn.Control.trim.Ki_lon_interp  SimulateUsing=Code generation
  Matrix Interpolation3 : simulink_extras/Additional Lookup Tables/Matrix Interpolation  InterpMethod=Linear  ExtrapMethod=Clip  InterpolateDimension=2  TableData=SimIn.Control.trim.Kx_lon_interp  SimulateUsing=Code generation
  Matrix Interpolation4 : simulink_extras/Additional Lookup Tables/Matrix Interpolation  InterpMethod=Linear  ExtrapMethod=Clip  InterpolateDimension=2  TableData=SimIn.Control.trim.F_lon_interp  SimulateUsing=Code generation
  Matrix Interpolation5 : simulink_extras/Additional Lookup Tables/Matrix Interpolation  InterpMethod=Linear  ExtrapMethod=Clip  InterpolateDimension=2  TableData=SimIn.Control.trim.Ap_lon_interp  SimulateUsing=Code generation
  Matrix Interpolation6 : simulink_extras/Additional Lookup Tables/Matrix Interpolation  InterpMethod=Linear  ExtrapMethod=Clip  InterpolateDimension=2  TableData=SimIn.Control.trim.Bp_lon_interp  SimulateUsing=Code generation
  Matrix Interpolation8 : simulink_extras/Additional Lookup Tables/Matrix Interpolation  InterpMethod=Linear  ExtrapMethod=Clip  InterpolateDimension=2  TableData=SimIn.Control.trim.G_lon_interp  SimulateUsing=Code generation
  ctrl_sys_lon : Outport
  wires:
  f2/1 -> Matrix Interpolation6/4, Matrix Interpolation5/4, Matrix Interpolation16/4, Matrix Interpolation15/4, Matrix Interpolation14/4, Matrix Interpolation13/4, Matrix Interpolation8/4, Matrix Interpolation4/4, Matrix Interpolation12/4, Matrix Interpolation3/4, Matrix Interpolation2/4
  Bus Creator/1 -> ctrl_sys_lon/1  "ctrl_sys_lon"
  Matrix Interpolation12/1 -> Bus Creator/3  "Kv"
  Matrix Interpolation15/1 -> Bus Creator/8  "W"
  Matrix Interpolation5/1 -> Bus Creator/10  "Ap"
  Matrix Interpolation4/1 -> Bus Creator/4  "F"
  Matrix Interpolation14/1 -> Bus Creator/7  "Cv"
  Matrix Interpolation2/1 -> Bus Creator/1  "Ki"
  Matrix Interpolation16/1 -> Bus Creator/9  "B"
  Matrix Interpolation8/1 -> Bus Creator/5  "G"
  Matrix Interpolation13/1 -> Bus Creator/6  "C"
  Matrix Interpolation3/1 -> Bus Creator/2  "Kx"
  k1/1 -> Matrix Interpolation16/1, Matrix Interpolation6/1, Matrix Interpolation5/1, Matrix Interpolation15/1, Matrix Interpolation14/1, Matrix Interpolation13/1, Matrix Interpolation8/1, Matrix Interpolation4/1, Matrix Interpolation12/1, Matrix Interpolation3/1, Matrix Interpolation2/1
  k2/1 -> Matrix Interpolation6/3, Matrix Interpolation5/3, Matrix Interpolation16/3, Matrix Interpolation15/3, Matrix Interpolation14/3, Matrix Interpolation13/3, Matrix Interpolation8/3, Matrix Interpolation4/3, Matrix Interpolation12/3, Matrix Interpolation3/3, Matrix Interpolation2/3
  Matrix Interpolation6/1 -> Bus Creator/11  "Bp"
  f1/1 -> Matrix Interpolation6/2, Matrix Interpolation5/2, Matrix Interpolation16/2, Matrix Interpolation15/2, Matrix Interpolation14/2, Matrix Interpolation13/2, Matrix Interpolation8/2, Matrix Interpolation4/2, Matrix Interpolation12/2, Matrix Interpolation3/2, Matrix Interpolation2/2

== matlab function ComponentsLib/ConvertToControlFrame/MATLAB Function ==
  data: u input; y output double size=[4,1]
function y = fcn(u)

s = cos(u/2);
v = sin(u/2);
y = [s, 0*v, 0*v, v]';

== matlab function ComponentsLib/GeneratePseudoInverse ==
  data: W input; M output; B input
function M = fcn(W,B)

M = W\B'*inv(B*inv(W)*B');
